simulink model "ADP_based_square_formation_control"  (R2024a)
settings: Solver=VariableStepAuto  StartTime=0.0  StopTime=10  RelTol=1e-3
(part 1 of 2)
settings Model: Creator=LOQ  LastModifiedBy=LOQ

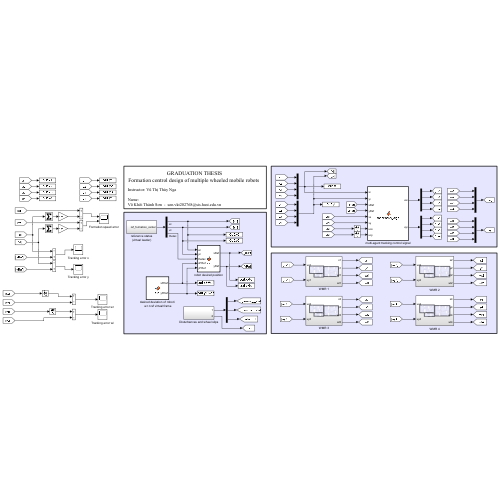
[thumbnail: Simulink's stored preview of the top-level diagram]
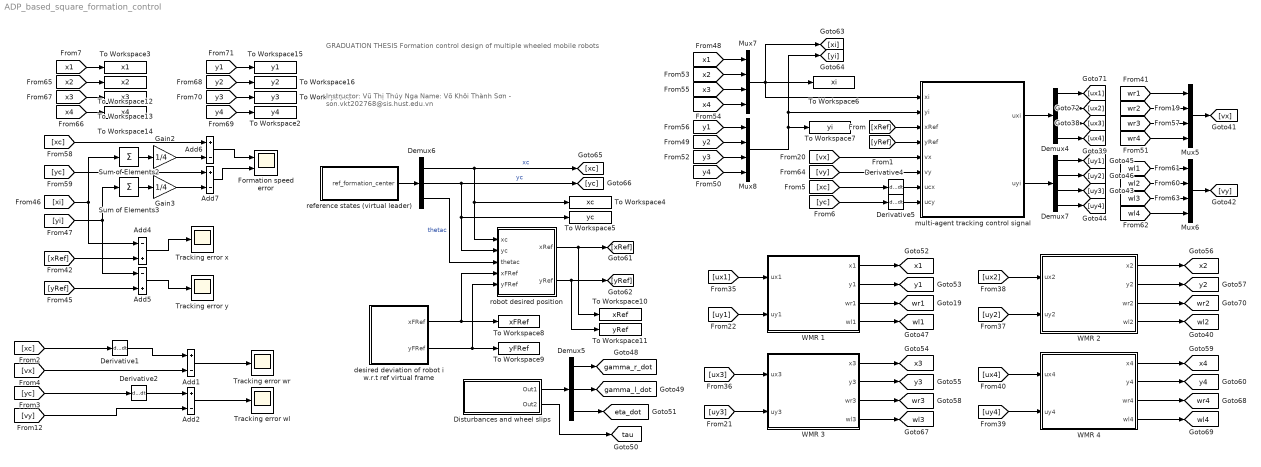
== system ADP_based_square_formation_control ==
  note: GRADUATION THESIS
      | Formation control design of multiple wheeled mobile robots
  note: Instructor: Vũ Thị Thúy Nga
      |
      | Name:
      | Võ Khôi Thành Sơn - son.vkt202768@sis.hust.edu.vn
  Add{1..2,6..7} (4 alike) : Sum  Inputs=+-
  Add4 : Sum  Inputs=-+
  Add5 : Sum  Inputs=-+
  Demux4 : Demux
  Demux5 : Demux  Outputs=3
  Demux6 : Demux  Outputs=3
  Demux7 : Demux
  Derivative{1..2,4..5} (4 alike) : Derivative
  Disturbances and wheel slips : Subsystem
  Formation speed error : Scope  NumInputPorts=2
  Gain2 : Gain  Gain=1/4
  Gain3 : Gain  Gain=1/4
  Mux{5..8} (4 alike) : Mux
  Sum of Elements2 : Sum  Inputs=+
  Sum of Elements3 : Sum  Inputs=+
  To Workspace1 : ToWorkspace  VariableName=y3  SampleTime=-1
  To Workspace10 : ToWorkspace  VariableName=xRef  SampleTime=-1
  To Workspace11 : ToWorkspace  VariableName=yRef  SampleTime=-1
  To Workspace12 : ToWorkspace  VariableName=x2  SampleTime=-1
  To Workspace13 : ToWorkspace  VariableName=x3  SampleTime=-1
  To Workspace14 : ToWorkspace  VariableName=x4  SampleTime=-1
  To Workspace15 : ToWorkspace  VariableName=y1  SampleTime=-1
  To Workspace16 : ToWorkspace  VariableName=y2  SampleTime=-1
  To Workspace2 : ToWorkspace  VariableName=y4  SampleTime=-1
  To Workspace3 : ToWorkspace  VariableName=x1  SampleTime=-1
  To Workspace4 : ToWorkspace  VariableName=xc  SampleTime=-1
  To Workspace5 : ToWorkspace  VariableName=yc  SampleTime=-1
  To Workspace6 : ToWorkspace  VariableName=xi  SampleTime=-1
  To Workspace7 : ToWorkspace  VariableName=yi  SampleTime=-1
  To Workspace8 : ToWorkspace  VariableName=xFRef  SampleTime=-1
  To Workspace9 : ToWorkspace  VariableName=yFRef  SampleTime=-1
  Tracking error wl : Scope
  Tracking error wr : Scope
  Tracking error x : Scope
  Tracking error y : Scope
  WMR 1 : Subsystem
  WMR 2 : Subsystem
  WMR 3 : Subsystem
  WMR 4 : Subsystem
  desired deviation of robot i w.r.t ref virtual frame : MATLAB Function  TreatAsAtomicUnit=on
  multi-agent tracking control signal : MATLAB Function  TreatAsAtomicUnit=on
  reference states (virtual leader) : Subsystem
  robot desired position : MATLAB Function  TreatAsAtomicUnit=on
  tag scope: eta_dot=global, gamma_l_dot=global, gamma_r_dot=global, tau=global, wl1=global, wl2=global, wl3=global, wl4=global, wr1=global, wr2=global, wr3=global, wr4=global, x1=global, x2=global, x3=global, x4=global, y1=global, y2=global, y3=global, y4=global
  wires:
  Demux6/3 -> robot desired position/3(thetac)  "thetac"
  reference states (virtual leader)/1(ref_formation_center) -> Demux6/1
  WMR 2/4(wl2) -> [wl2]
  Demux5/3 -> [eta_dot]
  Sum of Elements2/1 -> Gain2/1
  Sum of Elements3/1 -> Gain3/1
  Demux6/2 -> robot desired position/2(yc), To Workspace5/1, [yc]  "yc"
  Add5/1 -> Tracking error y/1
  Mux7/1 -> [xi], multi-agent tracking control signal/1(xi), To Workspace6/1
  [uy3] -> WMR 3/2(uy3)
  [y1] -> Mux8/1
  Gain2/1 -> Add6/2
  [wl3] -> Mux6/3
  robot desired position/2(yRef) -> [yRef], To Workspace11/1
  Demux7/4 -> [uy4]
  WMR 2/1(x2) -> [x2]
  [yRef] -> Add5/2
  [uy1] -> WMR 1/2(uy1)
  WMR 2/2(y2) -> [y2]
  desired deviation of robot i w.r.t ref virtual frame/2(yFRef) -> To Workspace9/1, robot desired position/5(yFRef)
  [uy4] -> WMR 4/2(uy4)
  [ux1] -> WMR 1/1(ux1)
  Demux4/2 -> [ux2]
  [wr4] -> Mux5/4
  multi-agent tracking control signal/1(uxi) -> Demux4/1
  robot desired position/1(xRef) -> [xRef], To Workspace10/1
  Add7/1 -> Formation speed error/2
  [xRef] -> Add4/2
  [yc] -> Add7/1
  Demux4/4 -> [ux4]
  [wl4] -> Mux6/4
  Demux6/1 -> [xc], robot desired position/1(xc), To Workspace4/1  "xc"
  [xc] -> Add6/1
  Derivative5/1 -> multi-agent tracking control signal/8(ucy)
  Demux4/3 -> [ux3]
  WMR 4/1(x4) -> [x4]
  Demux4/1 -> [ux1]
  WMR 1/2(y1) -> [y1]
  [wr1] -> Mux5/1
  [y2] -> Mux8/2
  Add4/1 -> Tracking error x/1
  [ux2] -> WMR 2/1(ux2)
  Derivative4/1 -> multi-agent tracking control signal/7(ucx)
  WMR 1/3(wr1) -> [wr1]
  Mux6/1 -> [vy]
  WMR 3/4(wl3) -> [wl3]
  [x2] -> Mux7/2
  [wl2] -> Mux6/2
  Mux5/1 -> [vx]
  [ux4] -> WMR 4/1(ux4)
  [xc] -> Derivative4/1
  WMR 3/1(x3) -> [x3]
  Add6/1 -> Formation speed error/1
  [wl1] -> Mux6/1
  [wr3] -> Mux5/3
  [vy] -> multi-agent tracking control signal/6(vy)
  Demux7/1 -> [uy1]
  [y4] -> Mux8/4
  [vx] -> multi-agent tracking control signal/5(vx)
  Demux5/1 -> [gamma_r_dot]
  multi-agent tracking control signal/2(uyi) -> Demux7/1
  WMR 3/3(wr3) -> [wr3]
  [yc] -> Derivative5/1
  [wr2] -> Mux5/2
  [ux3] -> WMR 3/1(ux3)
  Mux8/1 -> [yi], multi-agent tracking control signal/2(yi), To Workspace7/1
  [x4] -> Mux7/4
  Demux7/2 -> [uy2]
  [yi] -> Add5/1, Sum of Elements3/1
  [y3] -> Mux8/3
  WMR 4/3(wr4) -> [wr4]
  Disturbances and wheel slips/2(Out2) -> [tau]
  [x3] -> Mux7/3
  [xi] -> Sum of Elements2/1, Add4/1
  Disturbances and wheel slips/1(Out1) -> Demux5/1
  WMR 1/1(x1) -> [x1]
  WMR 4/4(wl4) -> [wl4]
  Demux7/3 -> [uy3]
  Demux5/2 -> [gamma_l_dot]
  Gain3/1 -> Add7/2
  [uy2] -> WMR 2/2(uy2)
  desired deviation of robot i w.r.t ref virtual frame/1(xFRef) -> To Workspace8/1, robot desired position/4(xFRef)
  WMR 2/3(wr2) -> [wr2]
  WMR 4/2(y4) -> [y4]
  WMR 1/4(wl1) -> [wl1]
  [x1] -> Mux7/1
  WMR 3/2(y3) -> [y3]
  [xRef] -> multi-agent tracking control signal/3(xRef)
  [yRef] -> multi-agent tracking control signal/4(yRef)
  [yc] -> Derivative2/1
  [xc] -> Derivative1/1
  Derivative1/1 -> Add1/1
  [vx] -> Add1/2
  Add1/1 -> Tracking error wr/1
  Derivative2/1 -> Add2/1
  [vy] -> Add2/2
  Add2/1 -> Tracking error wl/1
  [x3] -> To Workspace13/1
  [y4] -> To Workspace2/1
  [y3] -> To Workspace1/1
  [x1] -> To Workspace3/1
  [y2] -> To Workspace16/1
  [x4] -> To Workspace14/1
  [y1] -> To Workspace15/1
  [x2] -> To Workspace12/1

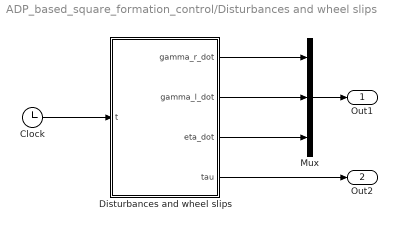
== system ADP_based_square_formation_control/Disturbances and wheel slips ==
  Clock : Clock
  Disturbances and wheel slips : MATLAB Function  TreatAsAtomicUnit=on
  Mux : Mux  Inputs=3
  Out1 : Outport
  Out2 : Outport  Port=2
  wires:
  Mux/1 -> Out1/1
  Clock/1 -> Disturbances and wheel slips/1(t)
  Disturbances and wheel slips/1(gamma_r_dot) -> Mux/1
  Disturbances and wheel slips/2(gamma_l_dot) -> Mux/2
  Disturbances and wheel slips/3(eta_dot) -> Mux/3
  Disturbances and wheel slips/4(tau) -> Out2/1

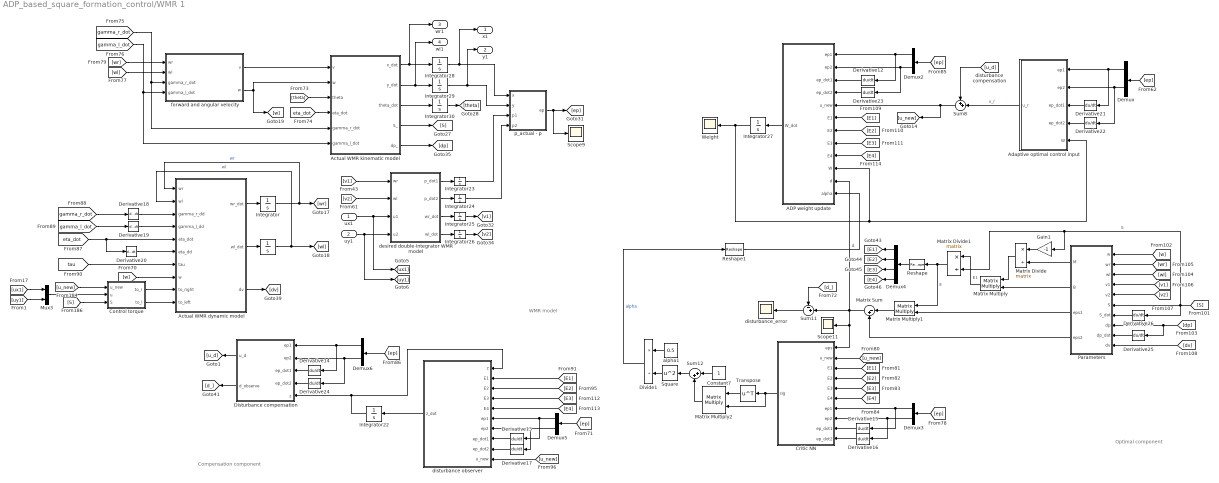
== system ADP_based_square_formation_control/WMR 1 ==
  note: WMR model
  note: Compensation component
  note: Optimal component
  ux1 : Inport
  uy1 : Inport  Port=2
  " " : Integrator
  ADP weight update : MATLAB Function  TreatAsAtomicUnit=on
  Actual WMR dynamic model : MATLAB Function  TreatAsAtomicUnit=on
  "Actual WMR kinematic model " : MATLAB Function  TreatAsAtomicUnit=on
  Adaptive optimal control input : MATLAB Function  TreatAsAtomicUnit=on
  Constant7 : Constant
  Control torque : MATLAB Function  TreatAsAtomicUnit=on
  Critic NN : MATLAB Function  TreatAsAtomicUnit=on
  Demux{,2..3,5..6} (5 alike) : Demux  Outputs=2
  Demux4 : Demux
  Derivative{12..26} (15 alike) : Derivative
  Disturbance compensation : MATLAB Function  TreatAsAtomicUnit=on
  Divide1 : Product  Inputs=*/
  Gain1 : Gain  Gain=-1
  Integrator : Integrator
  Integrator22 : Integrator  InitialCondition=[0;0;0;0]
  Integrator{23..26} (4 alike) : Integrator  InitialCondition=1
  Integrator27 : Integrator  InitialCondition=[1;1;1;1;1;1]
  Integrator28 : Integrator  InitialCondition=0.7
  Integrator29 : Integrator  InitialCondition=0.5
  Integrator30 : Integrator
  Matrix Sum : Sum  Inputs=|-+
  Matrix Divide : Product  Inputs=*/  Multiplication=Matrix(*)
  Matrix Divide1 : Product  Inputs=*/  Multiplication=Matrix(*)
  Matrix Multiply : Product  Multiplication=Matrix(*)
  Matrix Multiply1 : Product  Multiplication=Matrix(*)
  Matrix Multiply2 : Product  Multiplication=Matrix(*)
  Mux3 : Mux  Inputs=2
  Parameters : MATLAB Function  TreatAsAtomicUnit=on
  Reshape : Reshape
  Reshape1 : Reshape  OutputDimensionality=Customize  OutputDimensions=[1]
  Scope11 : Scope
  Scope9 : Scope
  Square : Math  Operator=square
  Sum11 : Sum  Inputs=-+|
  Sum12 : Sum  Inputs=|++
  Sum8 : Sum  Inputs=++|
  Transpose : Math  Operator=transpose
  Weight : Scope
  alpha1 : Constant  Value=0.5
  desired double-integrator WMR model : MATLAB Function  TreatAsAtomicUnit=on
  disturbance observer : MATLAB Function  TreatAsAtomicUnit=on
  disturbance_error : Scope
  "forward and angular velocity " : MATLAB Function  TreatAsAtomicUnit=on
  p_actual - p : MATLAB Function  TreatAsAtomicUnit=on
  x1 : Outport
  y1 : Outport  Port=2
  wr1 : Outport  Port=3
  wl1 : Outport  Port=4
  wires:
  [ep] -> Demux5/1
  [dv] -> Parameters/10(dv)
  Derivative21/1 -> Adaptive optimal control input/3(ep_dot1)
  "Actual WMR kinematic model "/2(y_dot) -> wl1/1, Integrator29/1
  [E2] -> Critic NN/4(E2)
  Disturbance compensation/1(u_d) -> [u_d]
  Demux6/2 -> Disturbance compensation/2(ep2), Derivative24/1
  [E2] -> disturbance observer/3(E2)
  [E1] -> disturbance observer/2(E1)
  [w] -> Parameters/1(w)
  Parameters/1(M) -> Matrix Divide/2
  Sum11/1 -> disturbance_error/1
  [ep] -> Demux/1
  [E3] -> disturbance observer/4(E3)
  [tau] -> Actual WMR dynamic model/7(tau)
  Derivative20/1 -> Actual WMR dynamic model/6(eta_dd)
  [dp] -> Parameters/8(dp), Derivative25/1
  [E1] -> Critic NN/3(E1)
  "forward and angular velocity "/2(w) -> [w], "Actual WMR kinematic model "/2(w)
  Reshape1/1 -> ADP weight update/12(alpha)
  [v2] -> Parameters/5(v2)
  [E4] -> Critic NN/6(E4)
  [E3] -> ADP weight update/8(E3)
  Integrator26/1 -> [v2]
  [theta] -> "Actual WMR kinematic model "/3(theta)
  Actual WMR dynamic model/1(wr_dot) -> Integrator/1
  Gain1/1 -> Matrix Divide/1
  [E1] -> ADP weight update/6(E1)
  Divide1/1 -> Reshape1/1  "alpha"
  Demux5/2 -> disturbance observer/7(ep2), Derivative17/1
  alpha1/1 -> Divide1/1
  Critic NN/1(sig) -> Matrix Multiply2/2, Transpose/1
  [E3] -> Critic NN/5(E3)
  Matrix Multiply2/1 -> Sum12/2
  Constant7/1 -> Sum12/1
  Transpose/1 -> Matrix Multiply2/1
  "Actual WMR kinematic model "/1(x_dot) -> wr1/1, Integrator28/1
  Demux3/2 -> Derivative16/1, Critic NN/8(ep2)
  [E4] -> ADP weight update/9(E4)
  Demux4/1 -> [E1]
  [ep] -> Demux3/1
  Demux3/1 -> Critic NN/7(ep1), Derivative15/1
  [gamma_r_dot] -> Derivative18/1
  Demux4/3 -> [E3]
  [u_new] -> Critic NN/2(u_new)
  [wr] -> Parameters/2(wr)
  desired double-integrator WMR model/4(wl_dot) -> Integrator26/1
  Demux4/4 -> [E4]
  Demux4/2 -> [E2]
  Parameters/3(eps1) -> Matrix Multiply1/2
  Parameters/4(eps2) -> Matrix Sum/2
  "Actual WMR kinematic model "/4(S_) -> [S]
  [wr] -> "forward and angular velocity "/1(wr)
  Adaptive optimal control input/1(u_r) -> Sum8/2  "u_r"
  Derivative19/1 -> Actual WMR dynamic model/4(gamma_l_dd)
  Derivative26/1 -> Parameters/7(S_dot)
  [v1] -> Parameters/4(v1)
  Demux2/2 -> Derivative23/1, ADP weight update/2(ep2)
  Matrix Divide1/1 -> Matrix Multiply1/1, Reshape/1  "E"
  [wl] -> Parameters/3(wl)
  Matrix Multiply/1 -> Matrix Divide1/1  "E1"
  [E2] -> ADP weight update/7(E2)
  [u_new] -> disturbance observer/10(u_new)
  Disturbance compensation/2(d_observe) -> [d_]
  [gamma_l_dot] -> Derivative19/1
  Derivative24/1 -> Disturbance compensation/4(ep_dot2)
  "Actual WMR kinematic model "/5(dp_) -> [dp]
  Derivative13/1 -> disturbance observer/8(ep_dot1)
  Derivative22/1 -> Adaptive optimal control input/4(ep_dot2)
  Demux2/1 -> Derivative12/1, ADP weight update/1(ep1)
  Sum12/1 -> Square/1
  [E4] -> disturbance observer/5(E4)
  Derivative12/1 -> ADP weight update/3(ep_dot1)
  Derivative23/1 -> ADP weight update/4(ep_dot2)
  Demux/1 -> Derivative21/1, Adaptive optimal control input/1(ep1)
  [gamma_l_dot] -> "Actual WMR kinematic model "/6(gamma_l_dot), "forward and angular velocity "/4(gamma_l_dot)
  Integrator25/1 -> [v1]
  Square/1 -> Divide1/2
  [v1] -> desired double-integrator WMR model/1(wr)
  Integrator28/1 -> x1/1, p_actual - p/1(x)
  [gamma_r_dot] -> "Actual WMR kinematic model "/5(gamma_r_dot), "forward and angular velocity "/3(gamma_r_dot)
  [ep] -> Demux2/1
  Derivative17/1 -> disturbance observer/9(ep_dot2)
  desired double-integrator WMR model/2(p_dot2) -> Integrator24/1
  desired double-integrator WMR model/1(p_dot1) -> Integrator23/1
  Derivative16/1 -> Critic NN/10(ep_dot2)
  Integrator30/1 -> [theta]
  Derivative18/1 -> Actual WMR dynamic model/3(gamma_r_dd)
  [eta_dot] -> "Actual WMR kinematic model "/4(eta_dot)
  disturbance observer/1(z_dot) -> Integrator22/1
  Integrator/1 -> Actual WMR dynamic model/1(wr), [wr]  "wr"
  [d_] -> Sum11/1
  "Actual WMR kinematic model "/3(theta_dot) -> Integrator30/1
  Demux/2 -> Derivative22/1, Adaptive optimal control input/2(ep2)
  Control torque/1(to_r) -> Actual WMR dynamic model/9(to_right)
  Matrix Divide/1 -> Matrix Multiply/1
  [u_new] -> Control torque/1(u_new)
  Matrix Sum/1 -> Critic NN/1(eps), Scope11/1, ADP weight update/11(d), Sum11/2  "d"
  Derivative25/1 -> Parameters/9(dp_dot)
  [wl] -> "forward and angular velocity "/2(wl)
  [S] -> Parameters/6(S), Derivative26/1, Gain1/1, Matrix Divide1/2  "S"
  Demux6/1 -> Derivative14/1, Disturbance compensation/1(ep1)
  [v2] -> desired double-integrator WMR model/2(wl)
  Reshape/1 -> Demux4/1
  [ep] -> Demux6/1
  Derivative15/1 -> Critic NN/9(ep_dot1)
  ADP weight update/1(W_dot) -> Integrator27/1
  p_actual - p/1(ep) -> Scope9/1, [ep]
  [eta_dot] -> Derivative20/1, Actual WMR dynamic model/5(eta_dot)
  Mux3/1 -> Control torque/2(u)
  Integrator22/1 -> disturbance observer/1(z), Disturbance compensation/5(z)
  Demux5/1 -> disturbance observer/6(ep1), Derivative13/1
  Sum8/1 -> [u_new], ADP weight update/5(u_new)
  [S] -> Control torque/3(S)
  Integrator24/1 -> p_actual - p/4(p2)
  "forward and angular velocity "/1(v) -> "Actual WMR kinematic model "/1(v)
  " "/1 -> Actual WMR dynamic model/2(wl), [wl]  "wl"
  Actual WMR dynamic model/3(dv) -> [dv]
  Matrix Multiply1/1 -> Matrix Sum/1
  Actual WMR dynamic model/2(wl_dot) -> " "/1
  Derivative14/1 -> Disturbance compensation/3(ep_dot1)
  Control torque/2(to_l) -> Actual WMR dynamic model/10(to_left)
  desired double-integrator WMR model/3(wr_dot) -> Integrator25/1
  Integrator23/1 -> p_actual - p/3(p1)
  Integrator27/1 -> Weight/1, ADP weight update/10(W), Adaptive optimal control input/5(W)
  [w] -> Actual WMR dynamic model/8(w)
  Parameters/2(B) -> Matrix Multiply/2
  Integrator29/1 -> y1/1, p_actual - p/2(y)
  uy1/1 -> [uy1], desired double-integrator WMR model/4(u2)
  ux1/1 -> [ux1], desired double-integrator WMR model/3(u1)
  [uy1] -> Mux3/2
  [ux1] -> Mux3/1
  [u_d] -> Sum8/1

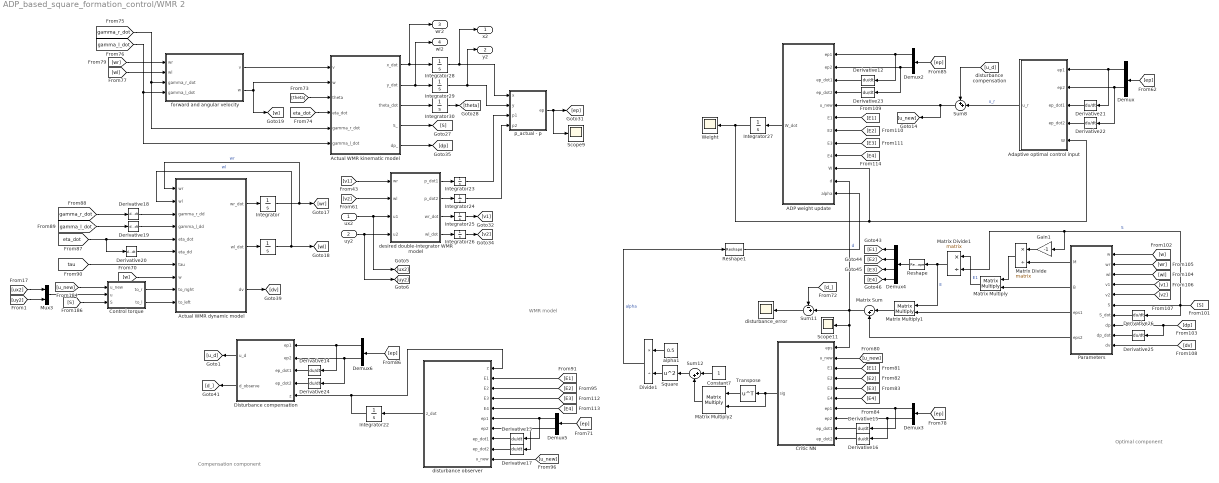
== system ADP_based_square_formation_control/WMR 2 ==
  note: Compensation component
  note: Optimal component
  note: WMR model
  ux2 : Inport
  uy2 : Inport  Port=2
  " " : Integrator
  ADP weight update : MATLAB Function  TreatAsAtomicUnit=on
  Actual WMR dynamic model : MATLAB Function  TreatAsAtomicUnit=on
  "Actual WMR kinematic model " : MATLAB Function  TreatAsAtomicUnit=on
  Adaptive optimal control input : MATLAB Function  TreatAsAtomicUnit=on
  Constant7 : Constant
  Control torque : MATLAB Function  TreatAsAtomicUnit=on
  Critic NN : MATLAB Function  TreatAsAtomicUnit=on
  Demux{,2..3,5..6} (5 alike) : Demux  Outputs=2
  Demux4 : Demux
  Derivative{12..26} (15 alike) : Derivative
  Disturbance compensation : MATLAB Function  TreatAsAtomicUnit=on
  Divide1 : Product  Inputs=*/
  Gain1 : Gain  Gain=-1
  Integrator : Integrator
  Integrator22 : Integrator  InitialCondition=[0;0;0;0]
  Integrator{23..26} (4 alike) : Integrator  InitialCondition=1
  Integrator27 : Integrator  InitialCondition=[1;1;1;1;1;1]
  Integrator28 : Integrator  InitialCondition=-0.6
  Integrator29 : Integrator  InitialCondition=0.4
  Integrator30 : Integrator  InitialCondition=pi/2
  Matrix Sum : Sum  Inputs=|-+
  Matrix Divide : Product  Inputs=*/  Multiplication=Matrix(*)
  Matrix Divide1 : Product  Inputs=*/  Multiplication=Matrix(*)
  Matrix Multiply : Product  Multiplication=Matrix(*)
  Matrix Multiply1 : Product  Multiplication=Matrix(*)
  Matrix Multiply2 : Product  Multiplication=Matrix(*)
  Mux3 : Mux  Inputs=2
  Parameters : MATLAB Function  TreatAsAtomicUnit=on
  Reshape : Reshape
  Reshape1 : Reshape  OutputDimensionality=Customize  OutputDimensions=[1]
  Scope11 : Scope
  Scope9 : Scope
  Square : Math  Operator=square
  Sum11 : Sum  Inputs=-+|
  Sum12 : Sum  Inputs=|++
  Sum8 : Sum  Inputs=++|
  Transpose : Math  Operator=transpose
  Weight : Scope
  alpha1 : Constant  Value=0.5
  desired double-integrator WMR model : MATLAB Function  TreatAsAtomicUnit=on
  disturbance observer : MATLAB Function  TreatAsAtomicUnit=on
  disturbance_error : Scope
  "forward and angular velocity " : MATLAB Function  TreatAsAtomicUnit=on
  p_actual - p : MATLAB Function  TreatAsAtomicUnit=on
  x2 : Outport
  y2 : Outport  Port=2
  wr2 : Outport  Port=3
  wl2 : Outport  Port=4
  wires:
  Integrator/1 -> Actual WMR dynamic model/1(wr), [wr]  "wr"
  Disturbance compensation/1(u_d) -> [u_d]
  [u_d] -> Sum8/1
  Actual WMR dynamic model/1(wr_dot) -> Integrator/1
  Constant7/1 -> Sum12/1
  [E4] -> disturbance observer/5(E4)
  Integrator23/1 -> p_actual - p/3(p1)
  [ux2] -> Mux3/1
  Reshape1/1 -> ADP weight update/12(alpha)
  Integrator24/1 -> p_actual - p/4(p2)
  Disturbance compensation/2(d_observe) -> [d_]
  Integrator29/1 -> y2/1, p_actual - p/2(y)
  [d_] -> Sum11/1
  [E3] -> Critic NN/5(E3)
  uy2/1 -> [uy2], desired double-integrator WMR model/4(u2)
  [ep] -> Demux3/1
  "Actual WMR kinematic model "/4(S_) -> [S]
  ux2/1 -> [ux2], desired double-integrator WMR model/3(u1)
  [w] -> Parameters/1(w)
  Matrix Multiply2/1 -> Sum12/2
  Control torque/1(to_r) -> Actual WMR dynamic model/9(to_right)
  Matrix Sum/1 -> Critic NN/1(eps), Scope11/1, ADP weight update/11(d), Sum11/2  "d"
  Parameters/2(B) -> Matrix Multiply/2
  Actual WMR dynamic model/2(wl_dot) -> " "/1
  Matrix Multiply1/1 -> Matrix Sum/1
  Demux5/1 -> disturbance observer/6(ep1), Derivative13/1
  Parameters/3(eps1) -> Matrix Multiply1/2
  Control torque/2(to_l) -> Actual WMR dynamic model/10(to_left)
  [E2] -> ADP weight update/7(E2)
  Integrator26/1 -> [v2]
  ADP weight update/1(W_dot) -> Integrator27/1
  [eta_dot] -> "Actual WMR kinematic model "/4(eta_dot)
  Integrator27/1 -> Weight/1, ADP weight update/10(W), Adaptive optimal control input/5(W)
  " "/1 -> Actual WMR dynamic model/2(wl), [wl]  "wl"
  Demux5/2 -> disturbance observer/7(ep2), Derivative17/1
  Demux2/2 -> Derivative23/1, ADP weight update/2(ep2)
  "Actual WMR kinematic model "/1(x_dot) -> wr2/1, Integrator28/1
  Actual WMR dynamic model/3(dv) -> [dv]
  [gamma_l_dot] -> "Actual WMR kinematic model "/6(gamma_l_dot), "forward and angular velocity "/4(gamma_l_dot)
  "forward and angular velocity "/1(v) -> "Actual WMR kinematic model "/1(v)
  p_actual - p/1(ep) -> Scope9/1, [ep]
  [gamma_r_dot] -> "Actual WMR kinematic model "/5(gamma_r_dot), "forward and angular velocity "/3(gamma_r_dot)
  Derivative23/1 -> ADP weight update/4(ep_dot2)
  [eta_dot] -> Derivative20/1, Actual WMR dynamic model/5(eta_dot)
  Matrix Divide/1 -> Matrix Multiply/1
  [S] -> Control torque/3(S)
  [ep] -> Demux6/1
  [S] -> Parameters/6(S), Derivative26/1, Gain1/1, Matrix Divide1/2  "S"
  Derivative12/1 -> ADP weight update/3(ep_dot1)
  [ep] -> Demux2/1
  Matrix Multiply/1 -> Matrix Divide1/1  "E1"
  Mux3/1 -> Control torque/2(u)
  Derivative14/1 -> Disturbance compensation/3(ep_dot1)
  Demux6/1 -> Derivative14/1, Disturbance compensation/1(ep1)
  Derivative17/1 -> disturbance observer/9(ep_dot2)
  Demux6/2 -> Disturbance compensation/2(ep2), Derivative24/1
  Reshape/1 -> Demux4/1
  Demux4/1 -> [E1]
  Divide1/1 -> Reshape1/1  "alpha"
  Demux/2 -> Derivative22/1, Adaptive optimal control input/2(ep2)
  [v1] -> desired double-integrator WMR model/1(wr)
  Integrator25/1 -> [v1]
  Gain1/1 -> Matrix Divide/1
  [u_new] -> Control torque/1(u_new)
  [u_new] -> Critic NN/2(u_new)
  Parameters/1(M) -> Matrix Divide/2
  Adaptive optimal control input/1(u_r) -> Sum8/2  "u_r"
  "Actual WMR kinematic model "/3(theta_dot) -> Integrator30/1
  Derivative18/1 -> Actual WMR dynamic model/3(gamma_r_dd)
  disturbance observer/1(z_dot) -> Integrator22/1
  Sum8/1 -> [u_new], ADP weight update/5(u_new)
  Integrator30/1 -> [theta]
  [w] -> Actual WMR dynamic model/8(w)
  Square/1 -> Divide1/2
  [wr] -> "forward and angular velocity "/1(wr)
  Derivative15/1 -> Critic NN/9(ep_dot1)
  desired double-integrator WMR model/4(wl_dot) -> Integrator26/1
  Demux/1 -> Derivative21/1, Adaptive optimal control input/1(ep1)
  Demux2/1 -> Derivative12/1, ADP weight update/1(ep1)
  Sum12/1 -> Square/1
  desired double-integrator WMR model/1(p_dot1) -> Integrator23/1
  [E1] -> ADP weight update/6(E1)
  Integrator28/1 -> x2/1, p_actual - p/1(x)
  [ep] -> Demux/1
  desired double-integrator WMR model/2(p_dot2) -> Integrator24/1
  Derivative19/1 -> Actual WMR dynamic model/4(gamma_l_dd)
  Demux3/1 -> Critic NN/7(ep1), Derivative15/1
  [u_new] -> disturbance observer/10(u_new)
  Derivative24/1 -> Disturbance compensation/4(ep_dot2)
  [E3] -> ADP weight update/8(E3)
  Derivative26/1 -> Parameters/7(S_dot)
  [v2] -> desired double-integrator WMR model/2(wl)
  [wl] -> Parameters/3(wl)
  Derivative22/1 -> Adaptive optimal control input/4(ep_dot2)
  Sum11/1 -> disturbance_error/1
  [E4] -> ADP weight update/9(E4)
  [uy2] -> Mux3/2
  Demux4/4 -> [E4]
  [wr] -> Parameters/2(wr)
  "forward and angular velocity "/2(w) -> [w], "Actual WMR kinematic model "/2(w)
  Demux3/2 -> Derivative16/1, Critic NN/8(ep2)
  Parameters/4(eps2) -> Matrix Sum/2
  Demux4/3 -> [E3]
  Demux4/2 -> [E2]
  [v2] -> Parameters/5(v2)
  [wl] -> "forward and angular velocity "/2(wl)
  [gamma_l_dot] -> Derivative19/1
  alpha1/1 -> Divide1/1
  Transpose/1 -> Matrix Multiply2/1
  [E3] -> disturbance observer/4(E3)
  [theta] -> "Actual WMR kinematic model "/3(theta)
  [v1] -> Parameters/4(v1)
  desired double-integrator WMR model/3(wr_dot) -> Integrator25/1
  Derivative20/1 -> Actual WMR dynamic model/6(eta_dd)
  Derivative16/1 -> Critic NN/10(ep_dot2)
  [tau] -> Actual WMR dynamic model/7(tau)
  [E4] -> Critic NN/6(E4)
  Derivative25/1 -> Parameters/9(dp_dot)
  [E1] -> Critic NN/3(E1)
  [dp] -> Parameters/8(dp), Derivative25/1
  Derivative21/1 -> Adaptive optimal control input/3(ep_dot1)
  [ep] -> Demux5/1
  [gamma_r_dot] -> Derivative18/1
  [dv] -> Parameters/10(dv)
  [E2] -> Critic NN/4(E2)
  Matrix Divide1/1 -> Matrix Multiply1/1, Reshape/1  "E"
  "Actual WMR kinematic model "/2(y_dot) -> wl2/1, Integrator29/1
  "Actual WMR kinematic model "/5(dp_) -> [dp]
  Integrator22/1 -> disturbance observer/1(z), Disturbance compensation/5(z)
  [E1] -> disturbance observer/2(E1)
  [E2] -> disturbance observer/3(E2)
  Critic NN/1(sig) -> Matrix Multiply2/2, Transpose/1
  Derivative13/1 -> disturbance observer/8(ep_dot1)

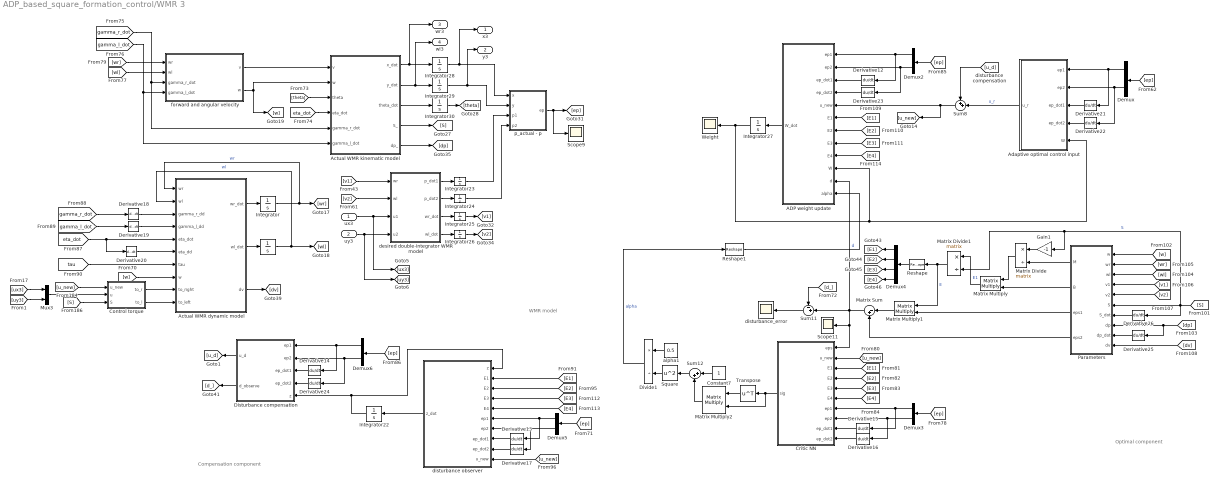
== system ADP_based_square_formation_control/WMR 3 ==
  note: Compensation component
  note: Optimal component
  note: WMR model
  ux3 : Inport
  uy3 : Inport  Port=2
  " " : Integrator
  ADP weight update : MATLAB Function  TreatAsAtomicUnit=on
  Actual WMR dynamic model : MATLAB Function  TreatAsAtomicUnit=on
  "Actual WMR kinematic model " : MATLAB Function  TreatAsAtomicUnit=on
  Adaptive optimal control input : MATLAB Function  TreatAsAtomicUnit=on
  Constant7 : Constant
  Control torque : MATLAB Function  TreatAsAtomicUnit=on
  Critic NN : MATLAB Function  TreatAsAtomicUnit=on
  Demux{,2..3,5..6} (5 alike) : Demux  Outputs=2
  Demux4 : Demux
  Derivative{12..26} (15 alike) : Derivative
  Disturbance compensation : MATLAB Function  TreatAsAtomicUnit=on
  Divide1 : Product  Inputs=*/
  Gain1 : Gain  Gain=-1
  Integrator : Integrator
  Integrator22 : Integrator  InitialCondition=[0;0;0;0]
  Integrator{23..26} (4 alike) : Integrator  InitialCondition=1
  Integrator27 : Integrator  InitialCondition=[1;1;1;1;1;1]
  Integrator28 : Integrator  InitialCondition=-0.8
  Integrator29 : Integrator  InitialCondition=0.3
  Integrator30 : Integrator  InitialCondition=-pi/3
  Matrix Sum : Sum  Inputs=|-+
  Matrix Divide : Product  Inputs=*/  Multiplication=Matrix(*)
  Matrix Divide1 : Product  Inputs=*/  Multiplication=Matrix(*)
  Matrix Multiply : Product  Multiplication=Matrix(*)
  Matrix Multiply1 : Product  Multiplication=Matrix(*)
  Matrix Multiply2 : Product  Multiplication=Matrix(*)
  Mux3 : Mux  Inputs=2
  Parameters : MATLAB Function  TreatAsAtomicUnit=on
  Reshape : Reshape
  Reshape1 : Reshape  OutputDimensionality=Customize  OutputDimensions=[1]
  Scope11 : Scope
  Scope9 : Scope
  Square : Math  Operator=square
  Sum11 : Sum  Inputs=-+|
  Sum12 : Sum  Inputs=|++
  Sum8 : Sum  Inputs=++|
  Transpose : Math  Operator=transpose
  Weight : Scope
  alpha1 : Constant  Value=0.5
  desired double-integrator WMR model : MATLAB Function  TreatAsAtomicUnit=on
  disturbance observer : MATLAB Function  TreatAsAtomicUnit=on
  disturbance_error : Scope
  "forward and angular velocity " : MATLAB Function  TreatAsAtomicUnit=on
  p_actual - p : MATLAB Function  TreatAsAtomicUnit=on
  x3 : Outport
  y3 : Outport  Port=2
  wr3 : Outport  Port=3
  wl3 : Outport  Port=4
  wires:
  Integrator/1 -> Actual WMR dynamic model/1(wr), [wr]  "wr"
  Disturbance compensation/1(u_d) -> [u_d]
  [u_d] -> Sum8/1
  Actual WMR dynamic model/1(wr_dot) -> Integrator/1
  Constant7/1 -> Sum12/1
  [E4] -> disturbance observer/5(E4)
  Integrator23/1 -> p_actual - p/3(p1)
  [ux3] -> Mux3/1
  Reshape1/1 -> ADP weight update/12(alpha)
  Integrator24/1 -> p_actual - p/4(p2)
  Disturbance compensation/2(d_observe) -> [d_]
  Integrator29/1 -> y3/1, p_actual - p/2(y)
  [d_] -> Sum11/1
  [E3] -> Critic NN/5(E3)
  uy3/1 -> [uy3], desired double-integrator WMR model/4(u2)
  [ep] -> Demux3/1
  "Actual WMR kinematic model "/4(S_) -> [S]
  ux3/1 -> [ux3], desired double-integrator WMR model/3(u1)
  [w] -> Parameters/1(w)
  Matrix Multiply2/1 -> Sum12/2
  Control torque/1(to_r) -> Actual WMR dynamic model/9(to_right)
  Matrix Sum/1 -> Critic NN/1(eps), Scope11/1, ADP weight update/11(d), Sum11/2  "d"
  Parameters/2(B) -> Matrix Multiply/2
  Actual WMR dynamic model/2(wl_dot) -> " "/1
  Matrix Multiply1/1 -> Matrix Sum/1
  Demux5/1 -> disturbance observer/6(ep1), Derivative13/1
  Parameters/3(eps1) -> Matrix Multiply1/2
  Control torque/2(to_l) -> Actual WMR dynamic model/10(to_left)
  [E2] -> ADP weight update/7(E2)
  Integrator26/1 -> [v2]
  ADP weight update/1(W_dot) -> Integrator27/1
  [eta_dot] -> "Actual WMR kinematic model "/4(eta_dot)
  Integrator27/1 -> Weight/1, ADP weight update/10(W), Adaptive optimal control input/5(W)
  " "/1 -> Actual WMR dynamic model/2(wl), [wl]  "wl"
  Demux5/2 -> disturbance observer/7(ep2), Derivative17/1
  Demux2/2 -> Derivative23/1, ADP weight update/2(ep2)
  "Actual WMR kinematic model "/1(x_dot) -> wr3/1, Integrator28/1
  Actual WMR dynamic model/3(dv) -> [dv]
  [gamma_l_dot] -> "Actual WMR kinematic model "/6(gamma_l_dot), "forward and angular velocity "/4(gamma_l_dot)
  "forward and angular velocity "/1(v) -> "Actual WMR kinematic model "/1(v)
  p_actual - p/1(ep) -> Scope9/1, [ep]
  [gamma_r_dot] -> "Actual WMR kinematic model "/5(gamma_r_dot), "forward and angular velocity "/3(gamma_r_dot)
  Derivative23/1 -> ADP weight update/4(ep_dot2)
  [eta_dot] -> Derivative20/1, Actual WMR dynamic model/5(eta_dot)
  Matrix Divide/1 -> Matrix Multiply/1
  [S] -> Control torque/3(S)
  [ep] -> Demux6/1
  [S] -> Parameters/6(S), Derivative26/1, Gain1/1, Matrix Divide1/2  "S"
  Derivative12/1 -> ADP weight update/3(ep_dot1)
  [ep] -> Demux2/1
  Matrix Multiply/1 -> Matrix Divide1/1  "E1"
  Mux3/1 -> Control torque/2(u)
  Derivative14/1 -> Disturbance compensation/3(ep_dot1)
  Demux6/1 -> Derivative14/1, Disturbance compensation/1(ep1)
  Derivative17/1 -> disturbance observer/9(ep_dot2)
  Demux6/2 -> Disturbance compensation/2(ep2), Derivative24/1
  Reshape/1 -> Demux4/1
  Demux4/1 -> [E1]
  Divide1/1 -> Reshape1/1  "alpha"
  Demux/2 -> Derivative22/1, Adaptive optimal control input/2(ep2)
  [v1] -> desired double-integrator WMR model/1(wr)
  Integrator25/1 -> [v1]
  Gain1/1 -> Matrix Divide/1
  [u_new] -> Control torque/1(u_new)
  [u_new] -> Critic NN/2(u_new)
  Parameters/1(M) -> Matrix Divide/2
  Adaptive optimal control input/1(u_r) -> Sum8/2  "u_r"
  "Actual WMR kinematic model "/3(theta_dot) -> Integrator30/1
  Derivative18/1 -> Actual WMR dynamic model/3(gamma_r_dd)
  disturbance observer/1(z_dot) -> Integrator22/1
  Sum8/1 -> [u_new], ADP weight update/5(u_new)
  Integrator30/1 -> [theta]
  [w] -> Actual WMR dynamic model/8(w)
  Square/1 -> Divide1/2
  [wr] -> "forward and angular velocity "/1(wr)
  Derivative15/1 -> Critic NN/9(ep_dot1)
  desired double-integrator WMR model/4(wl_dot) -> Integrator26/1
  Demux/1 -> Derivative21/1, Adaptive optimal control input/1(ep1)
  Demux2/1 -> Derivative12/1, ADP weight update/1(ep1)
  Sum12/1 -> Square/1
  desired double-integrator WMR model/1(p_dot1) -> Integrator23/1
  [E1] -> ADP weight update/6(E1)
  Integrator28/1 -> x3/1, p_actual - p/1(x)
  [ep] -> Demux/1
  desired double-integrator WMR model/2(p_dot2) -> Integrator24/1
  Derivative19/1 -> Actual WMR dynamic model/4(gamma_l_dd)
  Demux3/1 -> Critic NN/7(ep1), Derivative15/1
  [u_new] -> disturbance observer/10(u_new)
  Derivative24/1 -> Disturbance compensation/4(ep_dot2)
  [E3] -> ADP weight update/8(E3)
  Derivative26/1 -> Parameters/7(S_dot)
  [v2] -> desired double-integrator WMR model/2(wl)
  [wl] -> Parameters/3(wl)
  Derivative22/1 -> Adaptive optimal control input/4(ep_dot2)
  Sum11/1 -> disturbance_error/1
  [E4] -> ADP weight update/9(E4)
  [uy3] -> Mux3/2
  Demux4/4 -> [E4]
  [wr] -> Parameters/2(wr)
  "forward and angular velocity "/2(w) -> [w], "Actual WMR kinematic model "/2(w)
  Demux3/2 -> Derivative16/1, Critic NN/8(ep2)
  Parameters/4(eps2) -> Matrix Sum/2
  Demux4/3 -> [E3]
  Demux4/2 -> [E2]
  [v2] -> Parameters/5(v2)
  [wl] -> "forward and angular velocity "/2(wl)
  [gamma_l_dot] -> Derivative19/1
  alpha1/1 -> Divide1/1
  Transpose/1 -> Matrix Multiply2/1
  [E3] -> disturbance observer/4(E3)
  [theta] -> "Actual WMR kinematic model "/3(theta)
  [v1] -> Parameters/4(v1)
  desired double-integrator WMR model/3(wr_dot) -> Integrator25/1
  Derivative20/1 -> Actual WMR dynamic model/6(eta_dd)
  Derivative16/1 -> Critic NN/10(ep_dot2)
  [tau] -> Actual WMR dynamic model/7(tau)
  [E4] -> Critic NN/6(E4)
  Derivative25/1 -> Parameters/9(dp_dot)
  [E1] -> Critic NN/3(E1)
  [dp] -> Parameters/8(dp), Derivative25/1
  Derivative21/1 -> Adaptive optimal control input/3(ep_dot1)
  [ep] -> Demux5/1
  [gamma_r_dot] -> Derivative18/1
  [dv] -> Parameters/10(dv)
  [E2] -> Critic NN/4(E2)
  Matrix Divide1/1 -> Matrix Multiply1/1, Reshape/1  "E"
  "Actual WMR kinematic model "/2(y_dot) -> wl3/1, Integrator29/1
  "Actual WMR kinematic model "/5(dp_) -> [dp]
  Integrator22/1 -> disturbance observer/1(z), Disturbance compensation/5(z)
  [E1] -> disturbance observer/2(E1)
  [E2] -> disturbance observer/3(E2)
  Critic NN/1(sig) -> Matrix Multiply2/2, Transpose/1
  Derivative13/1 -> disturbance observer/8(ep_dot1)

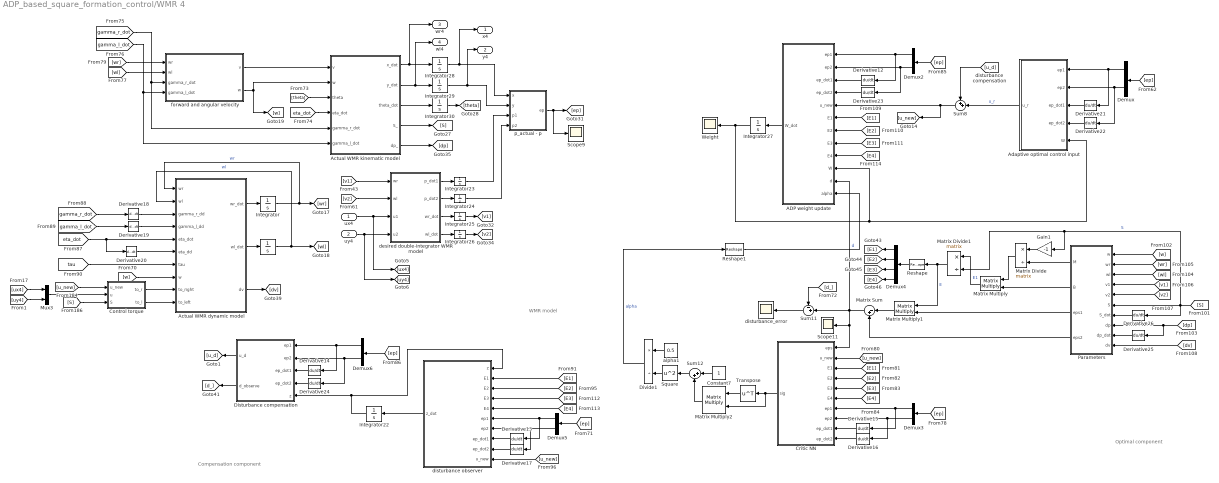
== system ADP_based_square_formation_control/WMR 4 ==
  note: Compensation component
  note: Optimal component
  note: WMR model
  ux4 : Inport
  uy4 : Inport  Port=2
  " " : Integrator
  ADP weight update : MATLAB Function  TreatAsAtomicUnit=on
  Actual WMR dynamic model : MATLAB Function  TreatAsAtomicUnit=on
  "Actual WMR kinematic model " : MATLAB Function  TreatAsAtomicUnit=on
  Adaptive optimal control input : MATLAB Function  TreatAsAtomicUnit=on
  Constant7 : Constant
  Control torque : MATLAB Function  TreatAsAtomicUnit=on
  Critic NN : MATLAB Function  TreatAsAtomicUnit=on
  Demux{,2..3,5..6} (5 alike) : Demux  Outputs=2
  Demux4 : Demux
  Derivative{12..26} (15 alike) : Derivative
  Disturbance compensation : MATLAB Function  TreatAsAtomicUnit=on
  Divide1 : Product  Inputs=*/
  Gain1 : Gain  Gain=-1
  Integrator : Integrator
  Integrator22 : Integrator  InitialCondition=[0;0;0;0]
  Integrator{23..26} (4 alike) : Integrator  InitialCondition=1
  Integrator27 : Integrator  InitialCondition=[1;1;1;1;1;1]
  Integrator28 : Integrator  InitialCondition=-0.5
  Integrator29 : Integrator  InitialCondition=0.9
  Integrator30 : Integrator  InitialCondition=pi/4
  Matrix Sum : Sum  Inputs=|-+
  Matrix Divide : Product  Inputs=*/  Multiplication=Matrix(*)
  Matrix Divide1 : Product  Inputs=*/  Multiplication=Matrix(*)
  Matrix Multiply : Product  Multiplication=Matrix(*)
  Matrix Multiply1 : Product  Multiplication=Matrix(*)
  Matrix Multiply2 : Product  Multiplication=Matrix(*)
  Mux3 : Mux  Inputs=2
  Parameters : MATLAB Function  TreatAsAtomicUnit=on
  Reshape : Reshape
  Reshape1 : Reshape  OutputDimensionality=Customize  OutputDimensions=[1]
  Scope11 : Scope
  Scope9 : Scope
  Square : Math  Operator=square
  Sum11 : Sum  Inputs=-+|
  Sum12 : Sum  Inputs=|++
  Sum8 : Sum  Inputs=++|
  Transpose : Math  Operator=transpose
  Weight : Scope
  alpha1 : Constant  Value=0.5
  desired double-integrator WMR model : MATLAB Function  TreatAsAtomicUnit=on
  disturbance observer : MATLAB Function  TreatAsAtomicUnit=on
  disturbance_error : Scope
  "forward and angular velocity " : MATLAB Function  TreatAsAtomicUnit=on
  p_actual - p : MATLAB Function  TreatAsAtomicUnit=on
  x4 : Outport
  y4 : Outport  Port=2
  wr4 : Outport  Port=3
  wl4 : Outport  Port=4
  wires:
  Integrator/1 -> Actual WMR dynamic model/1(wr), [wr]  "wr"
  Disturbance compensation/1(u_d) -> [u_d]
  [u_d] -> Sum8/1
  Actual WMR dynamic model/1(wr_dot) -> Integrator/1
  Constant7/1 -> Sum12/1
  [E4] -> disturbance observer/5(E4)
  Integrator23/1 -> p_actual - p/3(p1)
  [ux4] -> Mux3/1
  Reshape1/1 -> ADP weight update/12(alpha)
  Integrator24/1 -> p_actual - p/4(p2)
  Disturbance compensation/2(d_observe) -> [d_]
  Integrator29/1 -> y4/1, p_actual - p/2(y)
  [d_] -> Sum11/1
  [E3] -> Critic NN/5(E3)
  uy4/1 -> [uy4], desired double-integrator WMR model/4(u2)
  [ep] -> Demux3/1
  "Actual WMR kinematic model "/4(S_) -> [S]
  ux4/1 -> [ux4], desired double-integrator WMR model/3(u1)
  [w] -> Parameters/1(w)
  Matrix Multiply2/1 -> Sum12/2
  Control torque/1(to_r) -> Actual WMR dynamic model/9(to_right)
  Matrix Sum/1 -> Critic NN/1(eps), Scope11/1, ADP weight update/11(d), Sum11/2  "d"
  Parameters/2(B) -> Matrix Multiply/2
  Actual WMR dynamic model/2(wl_dot) -> " "/1
  Matrix Multiply1/1 -> Matrix Sum/1
  Demux5/1 -> disturbance observer/6(ep1), Derivative13/1
  Parameters/3(eps1) -> Matrix Multiply1/2
  Control torque/2(to_l) -> Actual WMR dynamic model/10(to_left)
  [E2] -> ADP weight update/7(E2)
  Integrator26/1 -> [v2]
  ADP weight update/1(W_dot) -> Integrator27/1
  [eta_dot] -> "Actual WMR kinematic model "/4(eta_dot)
  Integrator27/1 -> Weight/1, ADP weight update/10(W), Adaptive optimal control input/5(W)
  " "/1 -> Actual WMR dynamic model/2(wl), [wl]  "wl"
  Demux5/2 -> disturbance observer/7(ep2), Derivative17/1
  Demux2/2 -> Derivative23/1, ADP weight update/2(ep2)
  "Actual WMR kinematic model "/1(x_dot) -> wr4/1, Integrator28/1
  Actual WMR dynamic model/3(dv) -> [dv]
  [gamma_l_dot] -> "Actual WMR kinematic model "/6(gamma_l_dot), "forward and angular velocity "/4(gamma_l_dot)
  "forward and angular velocity "/1(v) -> "Actual WMR kinematic model "/1(v)
  p_actual - p/1(ep) -> Scope9/1, [ep]
  [gamma_r_dot] -> "Actual WMR kinematic model "/5(gamma_r_dot), "forward and angular velocity "/3(gamma_r_dot)
  Derivative23/1 -> ADP weight update/4(ep_dot2)
  [eta_dot] -> Derivative20/1, Actual WMR dynamic model/5(eta_dot)
  Matrix Divide/1 -> Matrix Multiply/1
  [S] -> Control torque/3(S)
  [ep] -> Demux6/1
  [S] -> Parameters/6(S), Derivative26/1, Gain1/1, Matrix Divide1/2  "S"
  Derivative12/1 -> ADP weight update/3(ep_dot1)
  [ep] -> Demux2/1
  Matrix Multiply/1 -> Matrix Divide1/1  "E1"
  Mux3/1 -> Control torque/2(u)
  Derivative14/1 -> Disturbance compensation/3(ep_dot1)
  Demux6/1 -> Derivative14/1, Disturbance compensation/1(ep1)
  Derivative17/1 -> disturbance observer/9(ep_dot2)
  Demux6/2 -> Disturbance compensation/2(ep2), Derivative24/1
  Reshape/1 -> Demux4/1
  Demux4/1 -> [E1]
  Divide1/1 -> Reshape1/1  "alpha"
  Demux/2 -> Derivative22/1, Adaptive optimal control input/2(ep2)
  [v1] -> desired double-integrator WMR model/1(wr)
  Integrator25/1 -> [v1]
  Gain1/1 -> Matrix Divide/1
  [u_new] -> Control torque/1(u_new)
  [u_new] -> Critic NN/2(u_new)
  Parameters/1(M) -> Matrix Divide/2
  Adaptive optimal control input/1(u_r) -> Sum8/2  "u_r"
  "Actual WMR kinematic model "/3(theta_dot) -> Integrator30/1
  Derivative18/1 -> Actual WMR dynamic model/3(gamma_r_dd)
  disturbance observer/1(z_dot) -> Integrator22/1
  Sum8/1 -> [u_new], ADP weight update/5(u_new)
  Integrator30/1 -> [theta]
  [w] -> Actual WMR dynamic model/8(w)
  Square/1 -> Divide1/2
  [wr] -> "forward and angular velocity "/1(wr)
  Derivative15/1 -> Critic NN/9(ep_dot1)
  desired double-integrator WMR model/4(wl_dot) -> Integrator26/1
  Demux/1 -> Derivative21/1, Adaptive optimal control input/1(ep1)
  Demux2/1 -> Derivative12/1, ADP weight update/1(ep1)
  Sum12/1 -> Square/1
  desired double-integrator WMR model/1(p_dot1) -> Integrator23/1
  [E1] -> ADP weight update/6(E1)
  Integrator28/1 -> x4/1, p_actual - p/1(x)
  [ep] -> Demux/1
  desired double-integrator WMR model/2(p_dot2) -> Integrator24/1
  Derivative19/1 -> Actual WMR dynamic model/4(gamma_l_dd)
  Demux3/1 -> Critic NN/7(ep1), Derivative15/1
  [u_new] -> disturbance observer/10(u_new)
  Derivative24/1 -> Disturbance compensation/4(ep_dot2)
  [E3] -> ADP weight update/8(E3)
  Derivative26/1 -> Parameters/7(S_dot)
  [v2] -> desired double-integrator WMR model/2(wl)
  [wl] -> Parameters/3(wl)
  Derivative22/1 -> Adaptive optimal control input/4(ep_dot2)
  Sum11/1 -> disturbance_error/1
  [E4] -> ADP weight update/9(E4)
  [uy4] -> Mux3/2
  Demux4/4 -> [E4]
  [wr] -> Parameters/2(wr)
  "forward and angular velocity "/2(w) -> [w], "Actual WMR kinematic model "/2(w)
  Demux3/2 -> Derivative16/1, Critic NN/8(ep2)
  Parameters/4(eps2) -> Matrix Sum/2
  Demux4/3 -> [E3]
  Demux4/2 -> [E2]
  [v2] -> Parameters/5(v2)
  [wl] -> "forward and angular velocity "/2(wl)
  [gamma_l_dot] -> Derivative19/1
  alpha1/1 -> Divide1/1
  Transpose/1 -> Matrix Multiply2/1
  [E3] -> disturbance observer/4(E3)
  [theta] -> "Actual WMR kinematic model "/3(theta)
  [v1] -> Parameters/4(v1)
  desired double-integrator WMR model/3(wr_dot) -> Integrator25/1
  Derivative20/1 -> Actual WMR dynamic model/6(eta_dd)
  Derivative16/1 -> Critic NN/10(ep_dot2)
  [tau] -> Actual WMR dynamic model/7(tau)
  [E4] -> Critic NN/6(E4)
  Derivative25/1 -> Parameters/9(dp_dot)
  [E1] -> Critic NN/3(E1)
  [dp] -> Parameters/8(dp), Derivative25/1
  Derivative21/1 -> Adaptive optimal control input/3(ep_dot1)
  [ep] -> Demux5/1
  [gamma_r_dot] -> Derivative18/1
  [dv] -> Parameters/10(dv)
  [E2] -> Critic NN/4(E2)
  Matrix Divide1/1 -> Matrix Multiply1/1, Reshape/1  "E"
  "Actual WMR kinematic model "/2(y_dot) -> wl4/1, Integrator29/1
  "Actual WMR kinematic model "/5(dp_) -> [dp]
  Integrator22/1 -> disturbance observer/1(z), Disturbance compensation/5(z)
  [E1] -> disturbance observer/2(E1)
  [E2] -> disturbance observer/3(E2)
  Critic NN/1(sig) -> Matrix Multiply2/2, Transpose/1
  Derivative13/1 -> disturbance observer/8(ep_dot1)

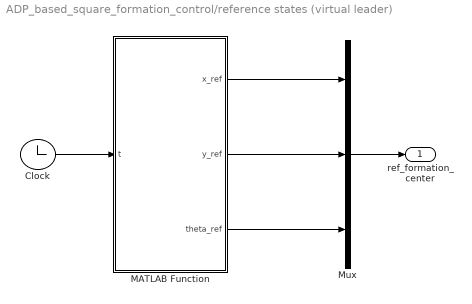
== system ADP_based_square_formation_control/reference states (virtual leader) ==
  Clock : Clock
  MATLAB Function : MATLAB Function  TreatAsAtomicUnit=on
  Mux : Mux  Inputs=3
  ref_formation_center : Outport
  wires:
  Mux/1 -> ref_formation_center/1
  Clock/1 -> MATLAB Function/1(t)
  MATLAB Function/1(x_ref) -> Mux/1
  MATLAB Function/2(y_ref) -> Mux/2
  MATLAB Function/3(theta_ref) -> Mux/3

== matlab function ADP_based_square_formation_control/WMR 3/Actual WMR kinematic model  ==
  data: v input; x_dot output; w input; theta input; y_dot output; theta_dot output; S_ output; eta_dot input; dp_ output; gamma_r_dot input; gamma_l_dot input
function [x_dot, y_dot, theta_dot, S_, dp_] = Kinematic (v,w,theta,eta_dot,gamma_r_dot,gamma_l_dot)

L = 0.6; % L =2b
r = 0.15; %m
a = 0.2; %m
% V: Robot velocity matrix
V = [v;w];

S = [cos(theta) -a*sin(theta);
     sin(theta) a*cos(theta);
      0 1];
dp = [-eta_dot*sin(theta);
       eta_dot*cos(theta);
       0];

% V = [wr;wl]
% S = [(r*cos(theta)/2)-(d*r*sin(theta)/L) (r*cos(theta)/2)+(d*r*sin(theta)/L);...
%      (r*sin(theta)/2)+(d*r*cos(theta)/L) (r*sin(theta)/2)-(d*r*cos(theta)/L);...
%       r/L -r/L];
% 
% dp = [(cos(theta)*(gamma_r_dot+gamma_l_dot)/2)-(d*sin(theta)*(gamma_r_dot-gamma_l_dot)/L)-eta_dot*sin(theta);
%       (sin(theta)*(gamma_r_dot+gamma_l_dot)/2)+(d*cos(theta)*(gamma_r_dot-gamma_l_dot)/L)+eta_dot*cos(theta);
%        (gamma_r_dot-gamma_l_dot)/L];

S_ = [(r*cos(theta)/2)-(a*r*sin(theta)/L) (r*cos(theta)/2)+(a*r*sin(theta)/L);
     (r*sin(theta)/2)+(a*r*cos(theta)/L) (r*sin(theta)/2)-(a*r*cos(theta)/L)];

dp_ = [(cos(theta)*(gamma_r_dot+gamma_l_dot)/2)-(a*sin(theta)*(gamma_r_dot-gamma_l_dot)/L)-eta_dot*sin(theta);
      (sin(theta)*(gamma_r_dot+gamma_l_dot)/2)+(a*cos(theta)*(gamma_r_dot-gamma_l_dot)/L)+eta_dot*cos(theta)];

% Output matrix
p_dot = S*V + dp;

% Output value 
x_dot = p_dot(1);
y_dot = p_dot(2);
theta_dot = p_dot(3);

end

== matlab function ADP_based_square_formation_control/WMR 3/Adaptive optimal control input ==
  data: u_r output; ep1 input; ep2 input; ep_dot1 input; ep_dot2 input; W input
function u_r  = control(ep1,ep2,ep_dot1,ep_dot2,W)

g_u = [0 0;
       0 0;
       1 0;
       0 1];    % 4x2
lambda = 2;

% x1 = ep;
% x2 = ep_dot+lambda*ep;

% x11 = x1(1);
% x12 = x1(2);   % When I add this the model failed to resolve although I don't use them for any calculation
% x21 = x2(1);
% x22 = x2(2);

% grad_vec = [2*x1(1) 0 0 0;
%             0 2*x1(2) 0 0;
%             x2(1) 0 x1(1) 0;
%             0 x2(2) 0 x1(2);
%             0 0 2*x2(1) 0;
%             0 0 0 2*x2(2)];   % 6x4

x11 = ep1;
x12 = ep2;
x21 = ep_dot1+lambda*ep1;
x22 = ep_dot2+lambda*ep2;
grad_vec = [2*x11 0 0 0;
            0 2*x12 0 0;
            x21 0 x11 0;
            0 x22 0 x12;
            0 0 2*x21 0;
            0 0 0 2*x22];   % 6x4

R = eye(2);

% Optimal control input
u_r = (-1/2)*R\(g_u')*grad_vec'*W;

end

== matlab function ADP_based_square_formation_control/WMR 3/Control torque ==
  data: u_new input; u input; to_r output; to_l output; S input
function [to_r,to_l] = fcn(u_new, u,S)
mG = 10; %kg
mW = 2; %kg
I_G = 4; %kgm^2
I_W = 0.1; %kgm^2
I_D = 0.05; %kgm^2
a = 0.2; %m
L = 0.6; %m
r = 0.15; %m

m11 = mG*(r^2/4 + a^2*r^2/(L^2)) + r^2*(I_G+2*I_D)/(L^2) + 2*mW*r^2 + I_W;
m12 = mG*(r^2/4 - a^2*r^2/(L^2)) - r^2*(I_G+2*I_D)/(L^2);
m21 = m12;
m22 = m11;
M = [m11 m12;
     m21 m22];

%% S*inv(M)*to-u = u_new
to = (M/S)*(u_new+u);   % to = M*inv(S)*(u_new+u)
to_r = to(1);
to_l = to(2);

end

== matlab function ADP_based_square_formation_control/WMR 3/Critic NN ==
  data: eps input; u_new input; E1 input; E2 input; E3 input; E4 input; ep1 input; sig output; ep2 input; ep_dot1 input; ep_dot2 input
function sig  = fcn(eps,u_new,E1,E2,E3,E4,ep1,ep2,ep_dot1,ep_dot2)
lambda = 2;
g_u = [0 0;
       0 0;
       1 0;
       0 1];    % 4x2
g_d = [0 0;
       0 0;
       1 0;
       0 1];    % 4x2

% x1 = ep;
% x2 = ep_dot+lambda*ep;
x11 = ep1;
x12 = ep2;
x21 = ep_dot1+lambda*ep1;
x22 = ep_dot2+lambda*ep2;

% % vec = [x1^2; x1*x2; x2^2];
% % grad_vec = [2*x1 0;      % 3x2
% %             x2 x1;
% %             0 2*x2];
grad_vec = [2*x11 0 0 0;
            0 2*x12 0 0;
            x21 0 x11 0;
            0 x22 0 x12;
            0 0 2*x21 0;
            0 0 0 2*x22];   % 6x4

% f = [x2-lambda*x1; E*x2-E*lambda*x1];   % 4x1
f = [x21-lambda*x11;
     x22-lambda*x12;
     E1*x21+E3*x22-(E1*lambda*x11+E3*lambda*x12);
     E2*x21+E4*x22-(E2*lambda*x11+E4*lambda*x12)]; 
% 
sig = grad_vec*(f + g_u*u_new + g_d*eps);   % 6x1
end

== matlab function ADP_based_square_formation_control/WMR 3/Disturbance compensation ==
  data: ep1 input; ep2 input; ep_dot1 input; ep_dot2 input; z input; u_d output; d_observe output
function [u_d, d_observe] = fcn(ep1,ep2,ep_dot1,ep_dot2,z)

lambda = 2;

x11 = ep1;
x12 = ep2;
x21 = ep_dot1+lambda*ep1;
x22 = ep_dot2+lambda*ep2;

% Disturbance observer
x = [x11;x12;x21;x22];
Lf = 30;
eps_ = z + Lf*x;

u_d = -eps_(3:4);

d_observe = eps_(3:4); % for plotting
end

== matlab function ADP_based_square_formation_control/WMR 3/Parameters ==
  data: M output; w input; B output; wr input; wl input; v1 input; v2 input; S input; S_dot input; dp input; dp_dot input; dv input; eps1 output; eps2 output
function [M,B,eps1,eps2] = fcn(w,wr,wl,v1,v2,S,S_dot,dp,dp_dot,dv)

mG = 10; %kg
mW = 2; %kg
I_G = 4; %kgm^2
I_W = 0.1; %kgm^2
I_D = 0.05; %kgm^2
a = 0.2; %m
L = 0.6; %m (L=2b)
r = 0.15; %m

m11 = mG*(r^2/4 + a^2*r^2/(L^2)) + r^2*(I_G+2*I_D)/(L^2) + 2*mW*r^2 + I_W;
m12 = mG*(r^2/4 - a^2*r^2/(L^2)) - r^2*(I_G+2*I_D)/(L^2);
m21 = m12;
m22 = m11;
M = [m11 m12;
     m21 m22];
B = mG*a*r^2/L*w*[0 1;-1 0];

V_actual = [wr;wl];
V = [v1;v2];
lambda = 2;

eps1 = dp-V;
eps2 = S*dv + S_dot*V_actual + dp_dot + lambda*S*V_actual + lambda*eps1;
% d = eps2 - E*eps1;    % 2x1

end

== matlab function ADP_based_square_formation_control/WMR 3/desired double-integrator WMR model ==
  data: wr input; p_dot1 output; wl input; p_dot2 output; wr_dot output; wl_dot output; u1 input; u2 input
function [p_dot1,p_dot2,wr_dot,wl_dot]  = fcn(wr,wl,u1,u2)
p_dot1 = wr;
p_dot2 = wl;
wr_dot = u1;
wl_dot = u2;

end

== matlab function ADP_based_square_formation_control/WMR 3/disturbance observer ==
  data: z input; E1 input; E2 input; E3 input; E4 input; ep1 input; ep2 input; ep_dot1 input; ep_dot2 input; u_new input; z_dot output
function z_dot = fcn(z,E1,E2,E3,E4,ep1,ep2,ep_dot1,ep_dot2,u_new)

lambda = 2;

x11 = ep1;
x12 = ep2;
x21 = ep_dot1+lambda*ep1;
x22 = ep_dot2+lambda*ep2;


% x = [x1;x2];   % 4x1
x = [x11;x12;x21;x22];
% f = [x2-lambda*x1; E*x2-E*lambda*x1];   % 4x1
f = [x21-lambda*x11;
     x22-lambda*x12;
     E1*x21+E3*x22-(E1*lambda*x11+E3*lambda*x12);
     E2*x21+E4*x22-(E2*lambda*x11+E4*lambda*x12)]; 
g_u = [0 0;
       0 0;
       1 0;
       0 1];    % 4x2
g_d = [0;
       0;
       1;
       1];    % 4x1

% Disturbance observer
Lf = 30;   
z_dot = -Lf*(g_d.*(z+Lf*x) + f + g_u*u_new); 

end

== matlab function ADP_based_square_formation_control/WMR 3/forward and angular velocity  ==
  data: wr input; v output; wl input; w output; gamma_r_dot input; gamma_l_dot input
function [v,w] = fcn(wr,wl, gamma_r_dot, gamma_l_dot)
L = 0.6; %m (L=2b)
r = 0.15; %m
v = r*(wr+wl)/2 + (gamma_r_dot+gamma_l_dot)/2;
w = r*(wr-wl)/L + (gamma_r_dot-gamma_l_dot)/L;

end

== matlab function ADP_based_square_formation_control/WMR 3/p_actual - p ==
  data: x input; ep output; y input; p1 input; p2 input
function ep = error(x,y,p1,p2)
ep1 = x-p1;
ep2 = y-p2;
ep = [ep1;ep2];
end

== matlab function ADP_based_square_formation_control/WMR 2/ADP weight update ==
  data: ep1 input; ep2 input; ep_dot1 input; ep_dot2 input; u_new input; E1 input; E2 input; E3 input; E4 input; W input; d input; alpha input; W_dot output
function W_dot = control(ep1,ep2,ep_dot1,ep_dot2,u_new,E1,E2,E3,E4,W,d,alpha)

lambda = 2;

g_u = [0 0;
       0 0;
       1 0;
       0 1];    % 4x2
g_d = [0 0;
       0 0;
       1 0;
       0 1];    % 4x2

% x1 = ep;
% x2 = ep_dot+lambda*ep;
x11 = ep1;
x12 = ep2;
x21 = ep_dot1+lambda*ep1;
x22 = ep_dot2+lambda*ep2;

% % vec = [x1^2; x1*x2; x2^2];
% % grad_vec = [2*x1 0;      % 3x2
% %             x2 x1;
% %             0 2*x2];
grad_vec = [2*x11 0 0 0;
            0 2*x12 0 0;
            x21 0 x11 0;
            0 x22 0 x12;
            0 0 2*x21 0;
            0 0 0 2*x22];   % 6x4
% 
% x = [x1;x2];   % 4x1
x = [x11;x12;x21;x22];

f = [x21-lambda*x11;
     x22-lambda*x12;
     E1*x21+E3*x22-(E1*lambda*x11+E3*lambda*x12);
     E2*x21+E4*x22-(E2*lambda*x11+E4*lambda*x12)]; 

sig = grad_vec*(f + g_u*u_new + g_d*d);   % 6x1

% Update weights
% alpha1 = 2;
alpha2 = 0.8;
Q = eye(4);
R = eye(2);

% W_dot = (-alpha1*sig*(sig'*W + x'*Q*x + u_new'*R*u_new))/((sig'*sig+1)^2) + (1/2)*alpha2*grad_vec*g_u/R *g_u'*x;

W_dot = -alpha*sig*(sig'*W + x'*Q*x + u_new'*R*u_new) + (1/2)*alpha2*grad_vec*g_u/R *g_u'*x;

end

== matlab function ADP_based_square_formation_control/WMR 2/Actual WMR dynamic model ==
  data: wr input; wl input; gamma_r_dd input; gamma_l_dd input; wr_dot output; eta_dot input; eta_dd input; tau input; w input; wl_dot output; dv output; to_right input; to_left input
function [wr_dot,wl_dot,dv]  = Dynamic(wr, wl, gamma_r_dd, gamma_l_dd, eta_dot, eta_dd, tau, w, to_right,to_left)
%% Parameters
mG = 10; %kg
mW = 2; %kg
I_G = 4; %kgm^2
I_W = 0.1; %kgm^2
I_D = 0.05; %kgm^2
a = 0.2; %m
L = 0.6; %m (L=2b)
r = 0.15; %m

m11 = mG*(r^2/4 + a^2*r^2/(L^2)) + r^2*(I_G+2*I_D)/(L^2) + 2*mW*r^2 + I_W;
m12 = mG*(r^2/4 - a^2*r^2/(L^2)) - r^2*(I_G+2*I_D)/(L^2);
m21 = m12;
m22 = m11;
M = [m11 m12;
     m21 m22];
B = mG*a*r^2/L*w*[0 1;-1 0];
Q1 = mG*r*(1+4*a^2/L^2)/4 + r*(I_G+2*I_D)/(2*L);
Q2 = mG*r*(1-4*a^2/L^2)/4 - r*(I_G+2*I_D)/(2*L);
Q = [Q1 Q2;
     Q2 Q1];
C = mG*(r/2)*w*[1;1];
G = mG*(a*r/L)*[1;-1];

gamma_dd = [gamma_r_dd; gamma_l_dd];

%% Dynamics of WMR
V = [wr;wl];
to = [to_right;to_left];
V_dot = (-M\B)*V + M\to - M\(Q*gamma_dd + C*eta_dot + G*eta_dd + tau);

wr_dot = V_dot(1);
wl_dot = V_dot(2);

dv = - M\(Q*gamma_dd + C*eta_dot + G*eta_dd + tau);

end
